simulink model "ros_with_simulink2014"  (Simulink 8.3)
settings: Solver=ode45  StartTime=0.0  StopTime=100  RelTol=1e-3
PreLoadFcn:
  | load center.mat;
  | Xref_ = center(1,:) * 43;
  | Yref_ = center(2,:) * 43;
  | 
  | Xref_ = Xref_ - Xref_(1);
  | Yref_ = Yref_ - Yref_(1);
  | 
  | Xref_ = Xref_(1,1:end);
  | Yref_ = Yref_(1,1:end);
  | 
  | N = size(Xref_);
  | N = N(2);
  | % Yref 世界坐标系 → frenet坐标系
  | [s_,rx,ry,rs,ryaw,rk] = convert_s(Xref_,Yref_);
  | rpath = [rx,ry,rs,ryaw,rk];
  | 
  | global v_acutal;
  | global deltaf_actual;
  | deltaf_actual = 0;
  | v_actual = 0;
undefined symbols (not defined in the file): Orientation, Position
libraries: robotlib x3, Solver_SF x1, simulink x1
settings Model: Creator=HY  LastModifiedBy=HY  CovModelRefEnable=off  CovSFcnEnable=on
settings DataIOCC: LimitDataPoints=off  SaveFormat=StructureWithTime  SignalLoggingSaveFormat=Dataset
settings DebuggingCC: UnderspecifiedInitializationDetection=Simplified  MergeDetectMultiDrivingBlocksExec=error  SolverPrmCheckMsg=none  FrameProcessingCompatibilityMsg=error  StateNameClashWarn=none
settings HardwareCC: ProdBitPerPointer=64  ProdLargestAtomicFloat=Float  ProdIntDivRoundTo=Zero  ProdEndianess=LittleEndian  ProdHWDeviceType=Specified
settings ModelReferenceCC: PropagateSignalLabelsOutOfModel=on
settings GRTTargetCC: CombineOutputUpdateFcns=on  GRTInterface=off

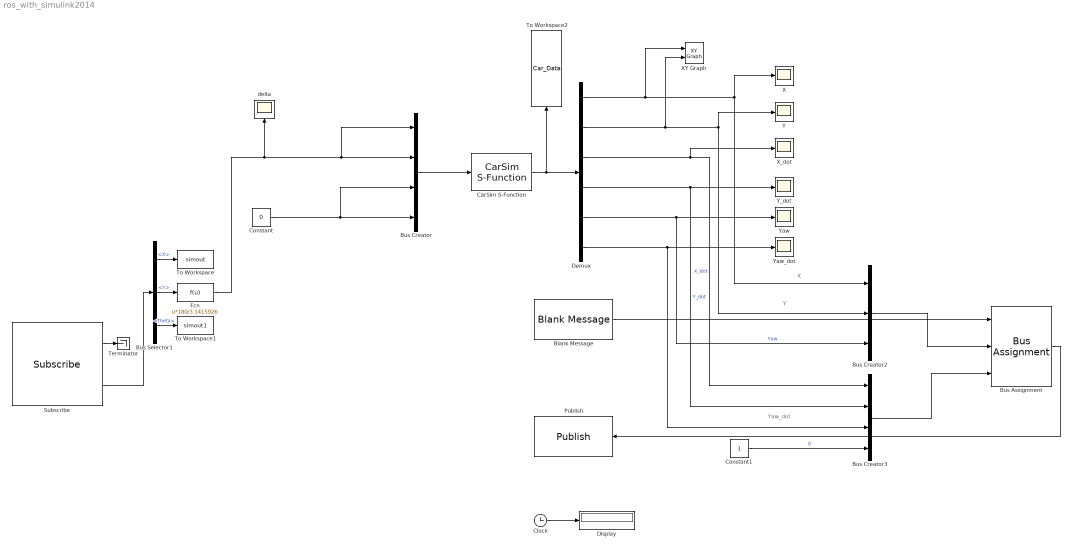
== system ros_with_simulink2014 ==
  note: Yaw_dot
  note: Y
  note: X
  Blank Message : robotlib/Blank Message  SourceLibraryInfo=This block requires Robotics System Toolbox  messageType=geometry_msgs/Pose  SampleTime=-1
  Bus Assignment : BusAssignment  AssignedSignals=Position,Orientation
  Bus Creator : BusCreator  Inputs=4
  Bus Creator2 : BusCreator  Inputs=3
  Bus Creator3 : BusCreator  Inputs=4
  Bus Selector1 : BusSelector  OutputSignals=X,Y,Theta
  CarSim S-Function : Solver_SF/CarSim S-Function  Priority=1  VehicleCode=i_i  SIMFILE=simfile
  Clock : Clock
  Constant : Constant  Value=0
  Constant1 : Constant
  Demux : Demux  Outputs=6
  Display : Display
  Fcn : Fcn  Expr=u*180/3.1415926
  Publish : robotlib/Publish  SourceLibraryInfo=This block requires Robotics System Toolbox  topicSource=Specify your own  topic=/simulink_pose  messageType=geometry_msgs/Pose  messageQueueLength=1
  Subscribe : robotlib/Subscribe  SourceLibraryInfo=This block requires Robotics System Toolbox  topicSource=Specify your own  topic=/control  messageType=geometry_msgs/Pose2D  sampleTime=-1  messageQueueLength=1
  Terminator : Terminator
  To Workspace : ToWorkspace  VariableName=simout  SaveFormat=Timeseries  SampleTime=-1
  To Workspace1 : ToWorkspace  VariableName=simout1  SaveFormat=Timeseries  SampleTime=-1
  To Workspace2 : ToWorkspace  VariableName=Car_Data  SaveFormat=Timeseries  SampleTime=-1
  X : Scope
      settings: TimeRange=auto  LimitDataPoints=on  MaxDataPoints=5000  SaveToWorkspace=off  SaveName=ScopeData  YMin=-42.71292  YMax=-12.50801  SampleTime=-1  DataFormat=Array
  XY Graph : simulink/Sinks/XY Graph  xmin=-20  xmax=150  ymin=-150  ymax=20  st=-1
  X_dot : Scope
      settings: TimeRange=auto  LimitDataPoints=on  MaxDataPoints=5000  SaveToWorkspace=off  SaveName=ScopeData2  YMin=-10  YMax=10  SampleTime=-1  DataFormat=Array
  Y : Scope
      settings: TimeRange=auto  LimitDataPoints=on  MaxDataPoints=5000  SaveToWorkspace=off  YMin=93.19739  YMax=109.62192  SampleTime=-1  DataFormat=Array
  Y_dot : Scope
      settings: TimeRange=auto  LimitDataPoints=on  MaxDataPoints=5000  SaveToWorkspace=off  SaveName=ScopeData3  YMin=10.00005  YMax=30.00005  SampleTime=-1  DataFormat=Array
  Yaw : Scope
      settings: TimeRange=auto  LimitDataPoints=on  MaxDataPoints=5000  SaveToWorkspace=off  SaveName=ScopeData4  YMin=47.29578  YMax=67.29578  SampleTime=-1  DataFormat=Array
  Yaw_dot : Scope
      settings: TimeRange=auto  LimitDataPoints=on  MaxDataPoints=5000  SaveToWorkspace=off  YMin=-10  YMax=10  SampleTime=-1  DataFormat=Array
  delta : Scope
      settings: TimeRange=auto  LimitDataPoints=on  MaxDataPoints=5000  SaveToWorkspace=off  YMin=-46.19472  YMax=14.68204  SampleTime=-1  DataFormat=Array
  wires:
  Subscribe/2 -> Bus Selector1/1
  Bus Assignment/1 -> Publish/1
  CarSim S-Function/1 -> Demux/1, To Workspace2/1
  Clock/1 -> Display/1
  Subscribe/1 -> Terminator/1
  Blank Message/1 -> Bus Assignment/1
  Demux/1 -> XY Graph/1, Bus Creator2/1, X/1
  Demux/2 -> XY Graph/2, Bus Creator2/2, Y/1
  Demux/3 -> Bus Creator3/1, X_dot/1  "X_dot"
  Demux/5 -> Bus Creator2/3, Yaw/1  "Yaw"
  Demux/6 -> Bus Creator3/3, Yaw_dot/1
  Constant/1 -> Bus Creator/3, Bus Creator/4
  Bus Creator/1 -> CarSim S-Function/1
  Bus Selector1/2 -> Fcn/1  "<Y>"
  Fcn/1 -> delta/1, Bus Creator/1, Bus Creator/2
  Bus Selector1/1 -> To Workspace/1  "<X>"
  Bus Selector1/3 -> To Workspace1/1  "<Theta>"
  Demux/4 -> Bus Creator3/2, Y_dot/1  "Y_dot"
  Constant1/1 -> Bus Creator3/4  "0"
  Bus Creator2/1 -> Bus Assignment/2
  Bus Creator3/1 -> Bus Assignment/3
